simulink model "H1_Z"  (R2020b)
settings: Solver=VariableStepAuto  StartTime=0.0  StopTime=10.0  RelTol=1e-3
settings Model: Creator=intel  LastModifiedBy=intel
settings DataIOCC: SaveOutput=off  SaveTime=off

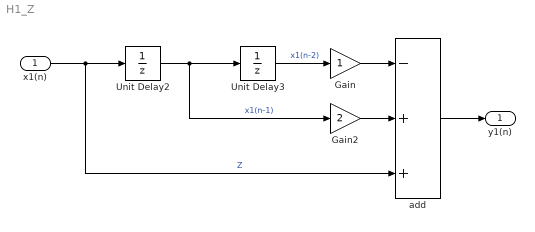
== system H1_Z ==
  x1(n) : Inport  OutDataTypeStr=double  PortDimensions=1  SampleTime=0
  Gain : Gain
  Gain2 : Gain  Gain=2
  Unit Delay2 : UnitDelay  SampleTime=-1  HasFrameUpgradeWarning=on
  Unit Delay3 : UnitDelay  SampleTime=-1  HasFrameUpgradeWarning=on
  add : Sum  Inputs=-++
  y1(n) : Outport  OutDataTypeStr=double  PortDimensions=1  SampleTime=0
  wires:
  x1(n)/1 -> add/3, Unit Delay2/1  "Z"
  Unit Delay2/1 -> Gain2/1, Unit Delay3/1  "x1(n-1)"
  Gain2/1 -> add/2
  Gain/1 -> add/1
  add/1 -> y1(n)/1
  Unit Delay3/1 -> Gain/1  "x1(n-2)"
